simulink model "un"  (R2020b)
settings: Solver=VariableStepAuto  StartTime=0.0  StopTime=50  RelTol=1e-3
values from neighbouring files (symbols this model uses):
  c1 = 1.2801    [input_1.m]
  c2 = 23.99    [input_1.m]
  c3 = 0.52    [input_1.m]
  c4 = 0.03    [input_1.m]
  fn = m*9.81    (= 3355.02)    [input_1.m]
  jw = 1.13    [input_1.m]
  kd = 5    [input_1.m]
  ki = 100000    [input_1.m]
  kp = 2500    [input_1.m]
  m = 342    [input_1.m]
  r = 0.33    [input_1.m]
  tb = 2000    [input_1.m]
libraries: pid_lib x1
settings Model: Creator=K E S SRINIVAS  LastModifiedBy=K E S SRINIVAS

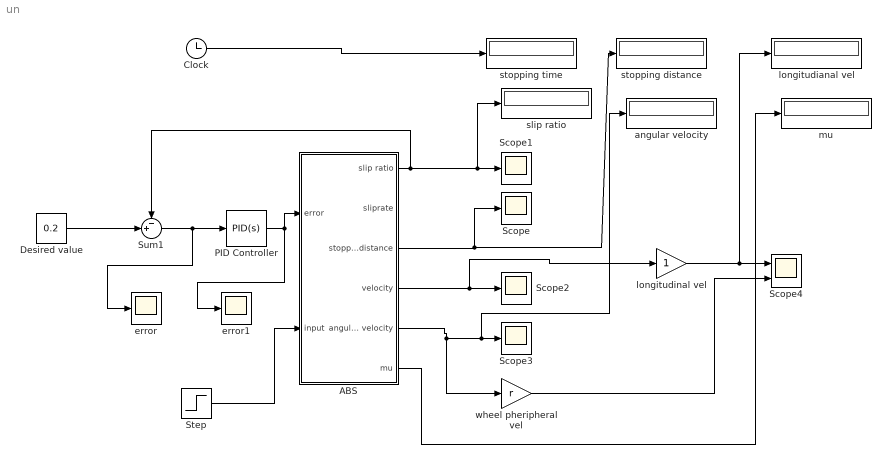
== system un ==
  ABS : Subsystem
  Clock : Clock
  Desired value : Constant  Value=0.2
  PID Controller : pid_lib/PID Controller  Controller=PID  Form=Parallel  TimeDomain=Continuous-time  UseExternalTs=off  SampleTime=-1  IntegratorMethod=Forward Euler  FilterMethod=Forward Euler  ControllerParametersSource=internal  P=kp  I=ki  D=kd  UseFilter=on  N=100  TunerSelectOption=Transfer Function Based (PID Tuner App)  InitialConditionSource=internal  InitialConditionForIntegrator=0  InitialConditionForFilter=0  DifferentiatorICPrevScaledInput=0  ExternalReset=none  TrackingMode=off  Kt=1  LimitOutput=off  SatLimitsSource=internal  UpperSaturationLimit=inf  LowerSaturationLimit=-inf  LinearizeAsGain=on  AntiWindupMode=none  Kb=1  POutMin=[]  POutMax=[]  IOutMin=[]  IOutMax=[]  DOutMin=[]  DOutMax=[]  NOutMin=[]  NOutMax=[]  SumOutMin=[]  SumOutMax=[]  SaturationOutMin=[]  SaturationOutMax=[]  PParamMin=[]  PParamMax=[]  IParamMin=[]  IParamMax=[]  DParamMin=[]  DParamMax=[]  NParamMin=[]  NParamMax=[]  KbParamMin=[]  KbParamMax=[]  KtParamMin=[]  KtParamMax=[]  KbOutMin=[]  KbOutMax=[]  KtOutMin=[]  KtOutMax=[]  IntegratorOutMin=[]  IntegratorOutMax=[]  FilterOutMin=[]  FilterOutMax=[]  SumI1OutMin=[]  SumI1OutMax=[]  SumI2OutMin=[]  SumI2OutMax=[]  SumI3OutMin=[]  SumI3OutMax=[]  SumI4OutMin=[]  SumI4OutMax=[]  SumDOutMin=[]  SumDOutMax=[]  DifferentiatorOutMin=[]  DifferentiatorOutMax=[]  FilterDiffOutCoefMin=[]  FilterDiffOutCoefMax=[]  ReciprocalOutMin=[]  ReciprocalOutMax=[]  SumDenOutMin=[]  SumDenOutMax=[]  SumNumOutMin=[]  SumNumOutMax=[]  DivideOutMin=[]  DivideOutMax=[]  UdiffTsProdOutMin=[]  UdiffTsProdOutMax=[]  NTsProdOutMin=[]  NTsProdOutMax=[]  UintegralTsProdOutMin=[]  UintegralTsProdOutMax=[]  UngainTsProdOutMin=[]  UngainTsProdOutMax=[]  IntegratorContinuousStateAttributes=''  IntegratorStateMustResolveToSignalObject=off  IntegratorRTWStateStorageClass=Auto  FilterContinuousStateAttributes=''  FilterStateMustResolveToSignalObject=off  FilterRTWStateStorageClass=Auto  ParallelPVariant=InternalParameters  IdealPVariant=Disabled  IVariant=InternalParameters  DVariant=InternalParameters  IntegratorVariant=Continuous  SatVariant=Disabled  AWVariant=Passthrough  PCopyVariant=Disabled  TRVariant=Disabled  FdbkBlocksVariant=Forward  IdealPFdbkVariant=Disabled  SatFdbkVariant=Disabled  DerivativeFilterVariant=ContFilter  NVariant=InternalParameters  NCopyVariant=Disabled  FilterICVariant=InternalICsFilter  IntegratorICVariant=InternalICs  ExternalResetVariant=Disabled  TRSumVariant=Passthrough  SumFdbkVariant=Disabled  SumVariant=Sum_PID  TsampFilterVariant=InternalTs  TsampNgainVariant=Passthrough  TsampIntegralVariant=Passthrough  ExternalSaturationOutDataTypeStr=Inherit: Same as second input
  Scope{,1..3} (4 alike) : Scope
  Scope4 : Scope  NumInputPorts=2
  Step : Step  After=tb  SampleTime=0
  Sum1 : Sum  Inputs=-+|
  angular velocity : Display
  error : Scope
  error1 : Scope
  longitudianal vel : Display
  longitudinal vel : Gain
  mu : Display
  slip ratio : Display
  stopping distance : Display
  stopping time : Display
  wheel pheripheral vel : Gain  Gain=r
  wires:
  ABS/1(slip ratio) -> Sum1/1, slip ratio/1, Scope1/1
  PID Controller/1 -> error1/1, ABS/1(error)
  Sum1/1 -> error/1, PID Controller/1
  Desired value/1 -> Sum1/2
  Clock/1 -> stopping time/1
  ABS/3(stopping distance) -> stopping distance/1, Scope/1
  ABS/4(velocity) -> longitudinal vel/1, Scope2/1
  ABS/5(angular velocity) -> wheel pheripheral vel/1, angular velocity/1, Scope3/1
  wheel pheripheral vel/1 -> Scope4/2
  ABS/6(mu) -> mu/1
  Step/1 -> ABS/2(input)
  longitudinal vel/1 -> Scope4/1, longitudianal vel/1

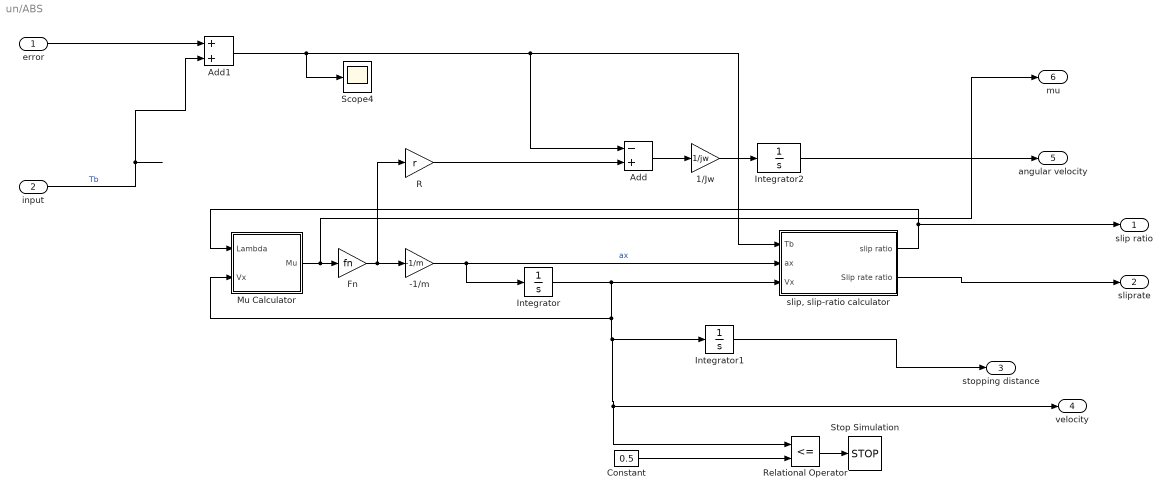
== system un/ABS ==
  error : Inport
  input : Inport  Port=2
  -1/m : Gain  Gain=-1/m
  1/Jw : Gain  Gain=1/jw
  Add : Sum  Inputs=-+
  Add1 : Sum
  Constant : Constant  Value=0.5
  Fn : Gain  Gain=fn
  Integrator : Integrator  InitialCondition=27.78  LimitOutput=on  LowerSaturationLimit=0
  Integrator1 : Integrator
  Integrator2 : Integrator  InitialCondition=84.18  LimitOutput=on  LowerSaturationLimit=0
  Mu Calculator : Subsystem
  R : Gain  Gain=r
  Relational Operator : RelationalOperator  Operator=<=  OutDataTypeStr=boolean  RndMeth=Simplest
  Scope4 : Scope
  Stop Simulation : Stop
  "slip, slip-ratio calculator" : Subsystem
  slip ratio : Outport
  sliprate : Outport  Port=2
  stopping distance : Outport  Port=3
  velocity : Outport  Port=4
  angular velocity : Outport  Port=5
  mu : Outport  Port=6
  wires:
  Mu Calculator/1(Mu) -> mu/1, Fn/1
  Integrator/1 -> velocity/1, Relational Operator/1, Integrator1/1, Mu Calculator/2(Vx), "slip, slip-ratio calculator"/3(Vx)
  -1/m/1 -> Integrator/1, "slip, slip-ratio calculator"/2(ax)  "ax"
  "slip, slip-ratio calculator"/1(slip ratio) -> Mu Calculator/1(Lambda), slip ratio/1
  Relational Operator/1 -> Stop Simulation/1
  Constant/1 -> Relational Operator/2
  Integrator1/1 -> stopping distance/1
  Add1/1 -> Scope4/1, Add/1, "slip, slip-ratio calculator"/1(Tb)
  Fn/1 -> R/1, -1/m/1
  R/1 -> Add/2
  Add/1 -> 1/Jw/1
  "slip, slip-ratio calculator"/2(Slip rate ratio) -> sliprate/1
  1/Jw/1 -> Integrator2/1
  Integrator2/1 -> angular velocity/1
  error/1 -> Add1/1
  input/1 -> Add1/2  "Tb"

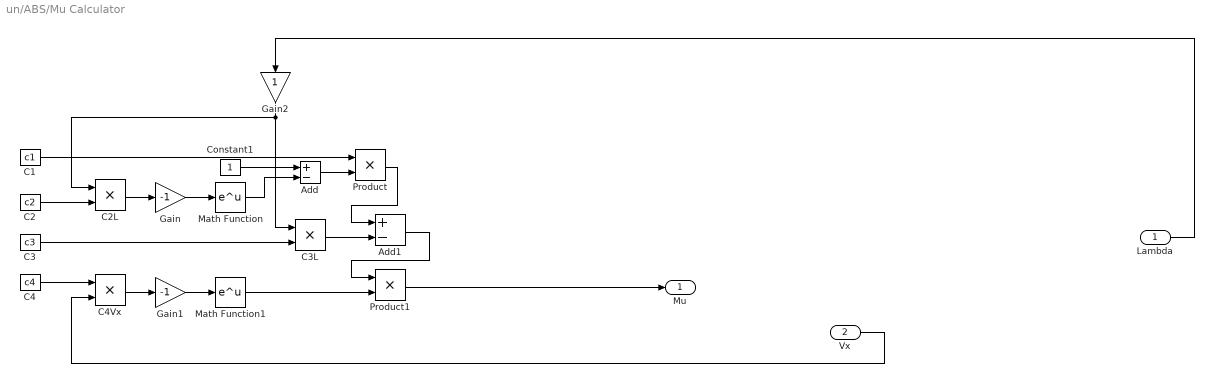
== system un/ABS/Mu Calculator ==
  Lambda : Inport
  Vx : Inport  Port=2
  Add : Sum  Inputs=+-
  Add1 : Sum  Inputs=+-
  C1 : Constant  Value=c1
  C2 : Constant  Value=c2
  C2L : Product
  C3 : Constant  Value=c3
  C3L : Product
  C4 : Constant  Value=c4
  C4Vx : Product
  Constant1 : Constant
  Gain : Gain  Gain=-1
  Gain1 : Gain  Gain=-1
  Gain2 : Gain
  Math Function : Math  SaturateOnIntegerOverflow=on
  Math Function1 : Math  SaturateOnIntegerOverflow=on
  Product : Product
  Product1 : Product
  Mu : Outport
  wires:
  C2/1 -> C2L/2
  Gain/1 -> Math Function/1
  C1/1 -> Product/1
  C2L/1 -> Gain/1
  Constant1/1 -> Add/1
  Vx/1 -> C4Vx/2
  C4/1 -> C4Vx/1
  Add/1 -> Product/2
  Math Function/1 -> Add/2
  Gain1/1 -> Math Function1/1
  Math Function1/1 -> Product1/2
  C3L/1 -> Add1/2
  Gain2/1 -> C3L/1, C2L/1
  Product1/1 -> Mu/1
  C4Vx/1 -> Gain1/1
  C3/1 -> C3L/2
  Product/1 -> Add1/1
  Add1/1 -> Product1/1
  Lambda/1 -> Gain2/1

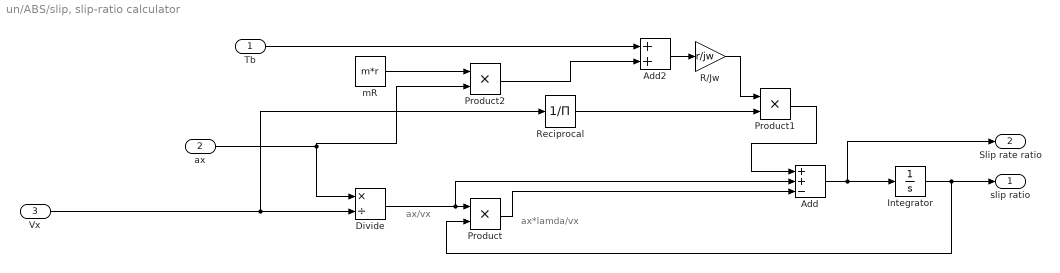
== system un/ABS/slip, slip-ratio calculator ==
  note: ax*lamda/vx
  note: ax/vx
  Tb : Inport
  ax : Inport  Port=2
  Vx : Inport  Port=3
  Add : Sum  Inputs=++-
  Add2 : Sum
  Divide : Product  Inputs=*/
  Integrator : Integrator  LimitOutput=on  UpperSaturationLimit=1  LowerSaturationLimit=0
  Product : Product
  Product1 : Product
  Product2 : Product
  R/Jw : Gain  Gain=r/jw
  Reciprocal : Product  Inputs=/
  mR : Constant  Value=m*r
  slip ratio : Outport
  Slip rate ratio : Outport  Port=2
  wires:
  ax/1 -> Divide/1, Product2/2
  Divide/1 -> Add/2, Product/1
  Product1/1 -> Add/1
  Product/1 -> Add/3
  Add/1 -> Slip rate ratio/1, Integrator/1
  R/Jw/1 -> Product1/1
  Tb/1 -> Add2/1
  Integrator/1 -> Product/2, slip ratio/1
  mR/1 -> Product2/1
  Product2/1 -> Add2/2
  Add2/1 -> R/Jw/1
  Vx/1 -> Reciprocal/1, Divide/2
  Reciprocal/1 -> Product1/2
